simulink model "combined_callback_csv_model_time"  (R2025b)
settings: Solver=FixedStepDiscrete  StartTime=0.0  StopTime=inf  FixedStep=0.1  RelTol=1e-3
PreLoadFcn:
  | callback_preload();
InitFcn:
  | callback_init();
StartFcn:
  | callback_start();
StopFcn:
  | callback_stop();
undefined symbols (not defined in the file or in its folder): amplitude_param, frequency_param, gain_param
CloseFcn:
  | callback_close();
settings Model: Creator=KoayXianCong  LastModifiedBy=KoayXianCong

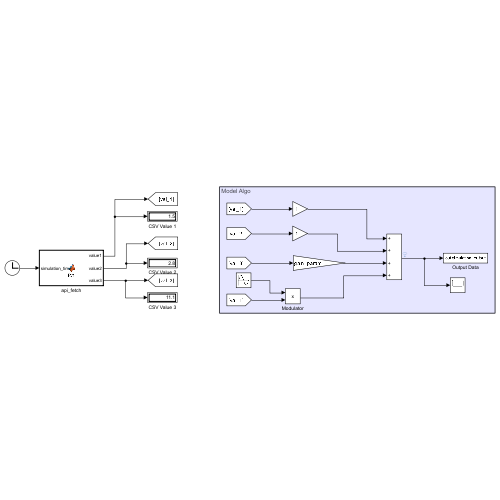
[thumbnail: Simulink's stored preview of the top-level diagram]
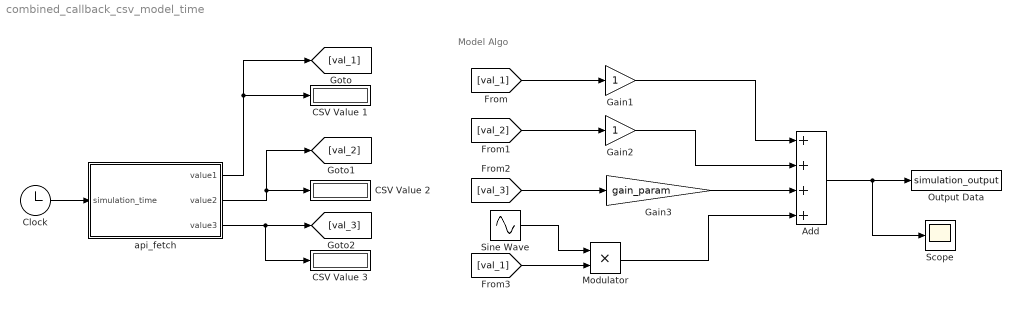
== system combined_callback_csv_model_time ==
  note: Model Algo
  Add : Sum  Inputs=++++
  CSV Value 1 : Display
  CSV Value 2 : Display
  CSV Value 3 : Display
  Clock : Clock
  Gain1 : Gain
  Gain2 : Gain
  Gain3 : Gain  Gain=gain_param
  Modulator : Product
  Output Data : ToWorkspace  VariableName=simulation_output  SampleTime=-1
  Scope : Scope
      settings: ActiveDisplayYMinimum=-6.0036548402670773  ActiveDisplayYMaximum=25.703654840267149
  Sine Wave : Sin  Amplitude=amplitude_param  Frequency=frequency_param  SampleTime=0
  api_fetch : MATLAB Function  TreatAsAtomicUnit=on
  wires:
  Sine Wave/1 -> Modulator/1
  [val_1] -> Modulator/2
  Clock/1 -> api_fetch/1(simulation_time)
  [val_1] -> Gain1/1
  api_fetch/2(value2) -> [val_2], CSV Value 2/1
  api_fetch/3(value3) -> [val_3], CSV Value 3/1
  [val_2] -> Gain2/1
  [val_3] -> Gain3/1
  api_fetch/1(value1) -> [val_1], CSV Value 1/1
  Gain1/1 -> Add/1
  Gain2/1 -> Add/2
  Gain3/1 -> Add/3
  Modulator/1 -> Add/4
  Add/1 -> Output Data/1, Scope/1

== matlab function combined_callback_csv_model_time/api_fetch ==
  data: simulation_time input; value1 output; value2 output; value3 output
function [value1, value2, value3] = fcn(simulation_time)                                                                                                                                       
% CSV Reader with Simulation Time                                                                                                                                                              
% Reads data from input_data.csv based on simulation time                                                                                                                                      
% Updates every 5.0 seconds of simulation time                                                                                                                                                 
                                                                                                                                                                                               
% Define update interval (in seconds)                                                                                                                                                          
UPDATE_INTERVAL = 5.0;  % Update every 5.0 seconds                                                                                                                                             
                                                                                                                                                                                               
% Declare persistent variables                                                                                                                                                                 
persistent lastUpdateTime;                                                                                                                                                                     
persistent data;                                                                                                                                                                               
                                                                                                                                                                                               
if isempty(lastUpdateTime)                                                                                                                                                                     
    lastUpdateTime = 0.0;  % Initialize last update time                                                                                                                                       
    data = [1.5, 1.8, 1.0];   % Default values                                                                                                                                                 
end                                                                                                                                                                                            
                                                                                                                                                                                               
% Update CSV data every UPDATE_INTERVAL seconds                                                                                                                                                
if simulation_time - lastUpdateTime >= UPDATE_INTERVAL                                                                                                                                         
    % Read CSV file using low-level file operations                                                                                                                                            
    newData = readCSVData();                                                                                                                                                                   
                                                                                                                                                                                               
    % Only update if valid data was received                                                                                                                                                   
    if ~all(isnan(newData)) && length(newData) >= 3                                                                                                                                            
        data = newData;                      % Update with new CSV data                                                                                                                        
    end                                                                                                                                                                                        
                                                                                                                                                                                               
    lastUpdateTime = simulation_time;  % Update with current time                                                                                                                              
end                                                                                                                                                                                            
                                                                                                                                                                                               
value1 = data(1);                                                                                                                                                                              
value2 = data(2);                                                                                                                                                                              
value3 = data(3);                                                                                                                                                                              
                                                                                                                                                                                               
end                                                                                                                                                                                            
                                                                                                                                                                                               
function data = readCSVData()                                                                                                                                                                  
% Internal function to read CSV data from input_data.csv                                                                                                                                       
data = [NaN, NaN, NaN];  % Default return value                                                                                                                                                
                                                                                                                                                                                               
% Attempt to open the CSV file (use 'r' instead of 'rt' for code generation)                                                                                                                                                                 
fid = fopen('input_data.csv', 'r');                                                                                                                                                           
if fid == -1                                                                                                                                                                                   
    return;                                                                                                                                                                                    
end                                                                                                                                                                                            
                                                                                                                                                                                               
% Read the first line                                                                                                                                                                          
line = fgets(fid);                                                                                                                                                                             
fclose(fid);                                                                                                                                                                                   
                                                                                                                                                                                               
% Check if fgets failed (returns -1) or line is empty
if ~ischar(line) || isempty(line)                                                                                                                                                                 
    return;                                                                                                                                                                                    
end                                                                                                                                                                                            
                                                                                                                                                                                               
% Parse the line manually to avoid table/readmatrix issues                                                                                                                                     
line = strtrim(line);                                                                                                                                                                          
% Split by comma                                                                                                                                                                               
parts = strsplit(line, ',');                                                                                                                                                                   
                                                                                                                                                                                               
% Convert each part to number                                                                                                                                                                  
data = zeros(1, length(parts));                                                                                                                                                                
for i = 1:length(parts)                                                                                                                                                                        
    numStr = strtrim(parts{i});                                                                                                                                                                
    tempVal = str2double(numStr);
    % Ensure the value is real (take real part if complex, or use NaN if invalid)
    if isnan(tempVal)
        data(i) = NaN;
    else
        data(i) = real(tempVal);
    end
end                                                                                                                                                                                            
                                                                                                                                                                                               
% Pad with default values if not enough values                                                                                                                                                 
if length(data) < 3                                                                                                                                                                            
    data = [data, 1.0 * ones(1, 3-length(data))];                                                                                                                                              
elseif length(data) > 3                                                                                                                                                                        
    data = data(1:3);                                                                                                                                                                          
end                                                                                                                                                                                            
                                                                                                                                                                                               
end
